simulink model "Model_3"  (R2020b)
settings: Solver=VariableStepAuto  StartTime=0.0  StopTime=25  RelTol=1e-3
settings Model: Creator=samar  LastModifiedBy=samar

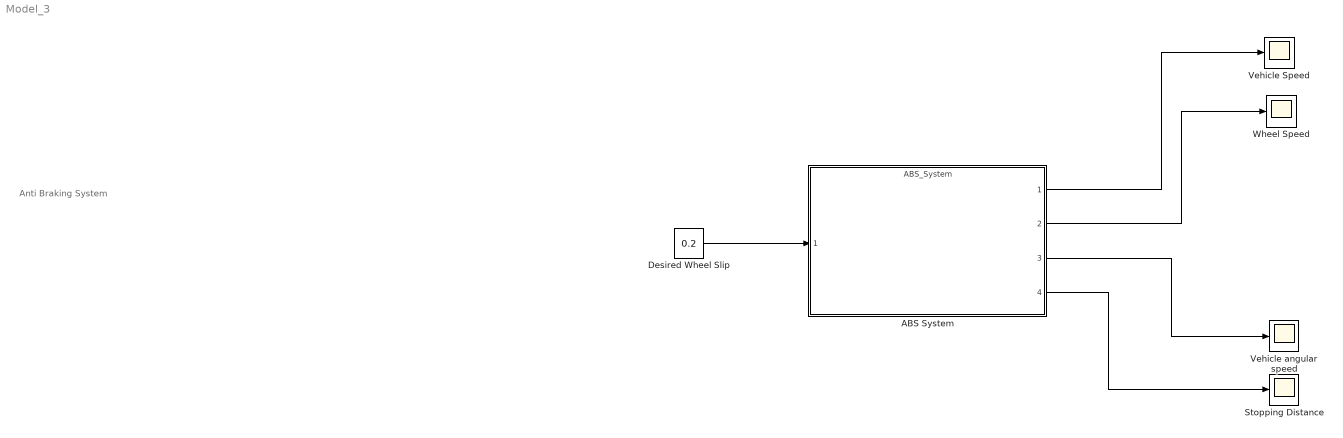
== system Model_3 ==
  note: Anti Braking System
  ABS System : ModelReference  ModelNameDialog=ABS_System  SimulationMode=Normal  ModelReferenceVersion=1.16
  Desired Wheel Slip : Constant  Value=0.2
  Stopping Distance : Scope
  Vehicle Speed : Scope
  Vehicle angular speed : Scope
  Wheel Speed : Scope
  wires:
  Desired Wheel Slip/1 -> ABS System/1
  ABS System/1 -> Vehicle Speed/1
  ABS System/2 -> Wheel Speed/1
  ABS System/3 -> Vehicle angular speed/1
  ABS System/4 -> Stopping Distance/1
